simulink model "Tipologia5_simulink"  (R2014a)
settings: Solver=ode45  StartTime=0.0  StopTime=10.0  RelTol=1e-3
libraries: cstblocks x2, simulink x1
settings Model: Creator=giova  LastModifiedBy=giova

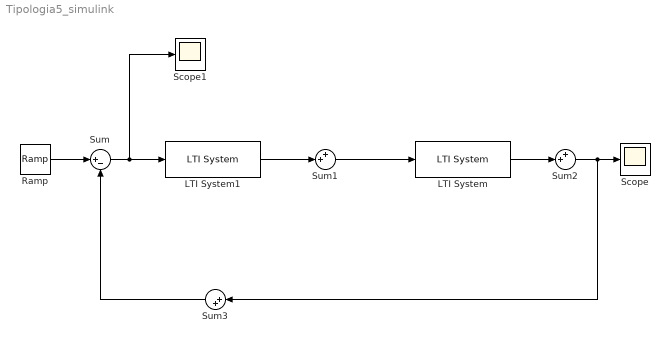
== system Tipologia5_simulink ==
  LTI System : cstblocks/LTI System  sys=F  IC=[]
  LTI System1 : cstblocks/LTI System  sys=C  IC=[]
  Ramp : simulink/Sources/Ramp  slope=1  start=0  X0=0
  Scope : Scope
  Scope1 : Scope
  Sum : Sum  Inputs=|+-
  Sum1 : Sum  Inputs=++|
  Sum2 : Sum  Inputs=++|
  Sum3 : Sum  Inputs=|++
  wires:
  LTI System/1 -> Sum2/2
  Sum1/1 -> LTI System/1
  LTI System1/1 -> Sum1/2
  Sum2/1 -> Sum3/1, Scope/1
  Ramp/1 -> Sum/1
  Sum/1 -> Scope1/1, LTI System1/1
  Sum3/1 -> Sum/2
